simulink model "albedo_test"  (R2023a)
settings: Solver=ode45  StartTime=0.0  StopTime=5.0  RelTol=1e-3  EnableMultiTasking=on
libraries: aausat3_lib x19
settings Model: Creator=kasperv  LastModifiedBy=jacobel-omar
settings SolverCC: AlgebraicLoopSolver=TrustRegion
settings DataIOCC: LimitDataPoints=on  SaveFormat=Array  SignalLoggingSaveFormat=ModelDataLogs  ReturnWorkspaceOutputs=off
settings OptimizationCC: ExpressionDepthLimit=2147483647  LifeSpan=inf
settings DebuggingCC: UnderspecifiedInitializationDetection=Classic  MergeDetectMultiDrivingBlocksExec=none  SolverPrmCheckMsg=warning  FcnCallInpInsideContextMsg=warning  UnconnectedInputMsg=warning  UnconnectedOutputMsg=warning  UnconnectedLineMsg=warning  StateNameClashWarn=warning  SFUnexpectedBacktrackingDiag=warning  SFNoUnconditionalDefaultTransitionDiag=warning  SFExecutionAtInitializationDiag=none  ArithmeticOperatorsInVariantConditions=warning
settings HardwareCC: ProdBitPerPointer=32  ProdBitPerSizeT=32  ProdBitPerPtrDiffT=32  ProdLargestAtomicFloat=None  ProdIntDivRoundTo=Undefined  ProdEndianess=Unspecified  ProdWordSize=32  ProdHWDeviceType=32-bit Generic
settings ModelReferenceCC: PropagateSignalLabelsOutOfModel=off
settings SFSimCC: SimUseLocalCustomCode=off  CustomCodeUndefinedFunction=UseInterfaceOnly
settings RTWCC: RTWUseLocalCustomCode=off
settings CodeAppCC: StateflowObjectComments=on
settings GRTTargetCC: TargetLangStandard=C89/C90 (ANSI)  CombineOutputUpdateFcns=off  GRTInterface=on
settings ConfigComp: CovMetricSettings=dw  CovSaveCumulativeToWorkspaceVar=on  CovSaveSingleToWorkspaceVar=on  CovExternalEMLEnable=off

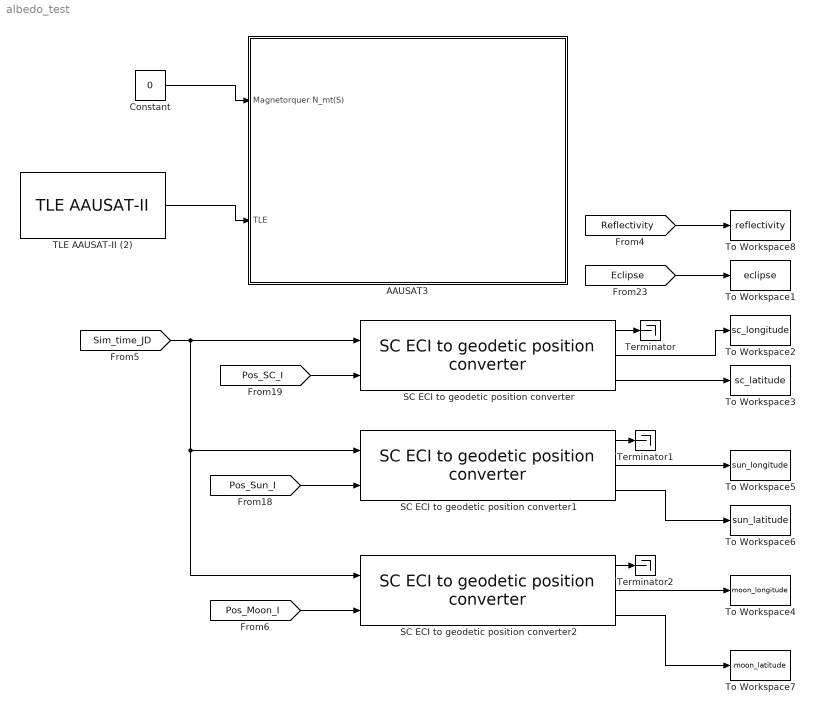
== system albedo_test ==
  AAUSAT3 : Subsystem  AncestorBlock=aausat3_lib/AAUSAT3  mask{r_com_s=[0.0493,0.0972,0.0549], sat_temp_start=293.15, mass_sc=0.7924, Dim=[0.1,0.2,0.1], inertia_c=[0.0017,0.0035,0.0036], init_jd=0, q_s_c=[0 0 0 1], q_init_I_S=[0 0 0 1], w_init_s=[0.1,0.1,0.1], Cd=2, rho=3.614e-14, solar_m_flux=4.5565e-6, solar_absorb_coeff=1.5, theta_e=65, refldata=load('lib/AlbedoToolbox-1.0/refl_data/2005/ga050101-051231'), redfac=1, Ts=1, enable_sensor_emulation=on, enable_env_disturbance=off}
      mask prompts: r_com_s "Center of Mass:"; sat_temp_start "Start Temperature of the Satellite [K]:"; mass_sc "Mass of the Satellite [kg]:"; Dim "Dimension of the Satellite [x,y,z][m];"; inertia_c "Inertia Matrix of the Satellite:"; init_jd "Initial time [JD]:"; q_s_c "Controller Reference Frame (S->C):"; q_init_I_S "Initial Attitude (I->S):"; w_init_s "Initial Angular Rate (S):"; Cd "Atmospheric Drag Coefficient [-]:"; rho "Atmospheric Density [kg/m^3]:"; solar_m_flux "Solar Momentum Flux [kg/ms^2]:"; solar_absorb_coeff "Solar Absorbtion Coefficient [-]:"; theta_e "Max. Angle of Theta [deg](eclipse: theta>r_earth/norm(R_SA)):"; refldata "Reflectivity Data (REFL Struct):"; redfac "Reduction Factor:"; Ts "Albedo Sampling Time [s]:"; enable_sensor_emulation "Enable Sensor Emulation."; enable_env_disturbance "Enable Environment Disturbance."
      mask Display:
      | image(imread('sat.jpg'));
      | color('w');
      | port_label('input', 1, 'N_mt(S)');
      | port_label('input', 2, 'TLE');
  Constant : Constant  Value=0
  SC ECI to geodetic position converter : aausat3_lib/Other Model Utilities/SC ECI to geodetic position converter
      settings: SourceProductName=AAUSAT3
  SC ECI to geodetic position converter1 : aausat3_lib/Other Model Utilities/SC ECI to geodetic position converter
      settings: SourceProductName=AAUSAT3
  SC ECI to geodetic position converter2 : aausat3_lib/Other Model Utilities/SC ECI to geodetic position converter
      settings: SourceProductName=AAUSAT3
  TLE AAUSAT-II (2) : aausat3_lib/Orbit and Ephemeris/TLE AAUSAT-II  satname='AAUSAT-II'  JulianDay=09321.69542252  xndt2o=0.00000555  xndd6o=0.0  bstar=.76898e-4  xincl=97.9251  xnodeo=24.1597  eo=0.0014245  omegao=254.1774  xmo=105.7862  xno=14.81823818  ts=1
      settings: SourceProductName=AAUSAT3
  Terminator : Terminator
  Terminator1 : Terminator
  Terminator2 : Terminator
  To Workspace1 : ToWorkspace  VariableName=eclipse  SampleTime=1
  To Workspace2 : ToWorkspace  VariableName=sc_longitude  SampleTime=1
  To Workspace3 : ToWorkspace  VariableName=sc_latitude  SampleTime=1
  To Workspace4 : ToWorkspace  VariableName=moon_longitude  SampleTime=1
  To Workspace5 : ToWorkspace  VariableName=sun_longitude  SampleTime=1
  To Workspace6 : ToWorkspace  VariableName=sun_latitude  SampleTime=1
  To Workspace7 : ToWorkspace  VariableName=moon_latitude  SampleTime=1
  To Workspace8 : ToWorkspace  VariableName=reflectivity  SampleTime=1
  wires:
  TLE AAUSAT-II (2)/1 -> AAUSAT3/2(TLE)
  Constant/1 -> AAUSAT3/1(Magnetorquer N_mt(S))
  [Eclipse] -> To Workspace1/1
  [Sim_time_JD] -> SC ECI to geodetic position converter/1, SC ECI to geodetic position converter1/1, SC ECI to geodetic position converter2/1
  [Pos_SC_I] -> SC ECI to geodetic position converter/2
  [Pos_Sun_I] -> SC ECI to geodetic position converter1/2
  SC ECI to geodetic position converter/1 -> Terminator/1
  SC ECI to geodetic position converter/2 -> To Workspace2/1
  SC ECI to geodetic position converter/3 -> To Workspace3/1
  SC ECI to geodetic position converter1/3 -> To Workspace6/1
  SC ECI to geodetic position converter1/2 -> To Workspace5/1
  SC ECI to geodetic position converter1/1 -> Terminator1/1
  [Pos_Moon_I] -> SC ECI to geodetic position converter2/2
  SC ECI to geodetic position converter2/3 -> To Workspace7/1
  SC ECI to geodetic position converter2/2 -> To Workspace4/1
  SC ECI to geodetic position converter2/1 -> Terminator2/1
  [Reflectivity] -> To Workspace8/1

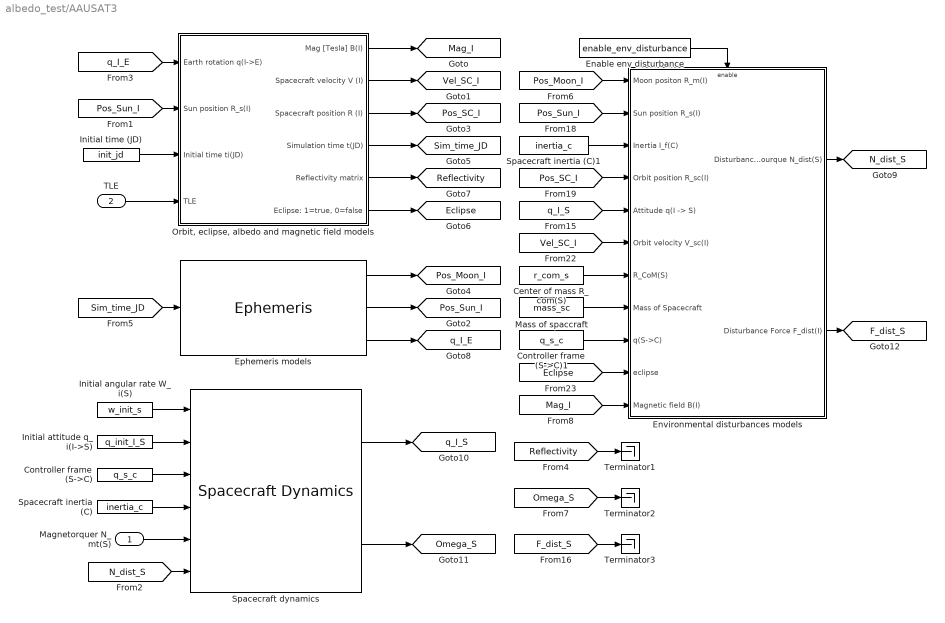
== system albedo_test/AAUSAT3 ==
  Magnetorquer N_mt(S) : Inport
  TLE : Inport  Port=2
  Center of mass R_com(S) : Constant  Value=r_com_s
  Controller frame (S->C) : Constant  Value=q_s_c
  Controller frame (S->C)1 : Constant  Value=q_s_c
  Enable env disturbance : Constant  Value=enable_env_disturbance
  Environmental disturbances models : Subsystem  AncestorBlock=aausat3_lib/Disturbances/Environment Disturbances  mask{Dim=Dim, sola_m_flux=solar_m_flux, solar_absorb_coeff=solar_absorb_coeff, rho=rho, Cd=Cd, G=6.672e-11, M_sun=1.989e30, M_earth=5.9742e24, M_moon=0.073483e24, enable_rad_dist=on, enable_atmospheric_dist=on, enable_gravity_dist=on, enable_mag_residual_dist=on}
      mask prompts: Dim "Satellite Dimension [x,y,z][m]:"; sola_m_flux "Solar Momentum Flux [kg/ms^2]:"; solar_absorb_coeff "Solar Absorbtion Coefficient [-]:"; rho "Atmospheric Density [kg/m^3]:"; Cd "Atmospheric Drag Coefficient [-]:"; G "Gravitational Constant [m^3/kgs^2]:"; M_sun "Mass of the Sun [kg]:"; M_earth "Mass of the Earth [kg]:"; M_moon "Mass of the Moon [kg]:"; enable_rad_dist "Enable Radiation Disturbanceses."; enable_atmospheric_dist "Enable Atmospheric Disturbanceses."; enable_gravity_dist "Enable Gravity Disturbanceses."; enable_mag_residual_dist "Enable Magnetic Residual Disturbance"
      mask help: Torque and force from the environment affecting the satellite.
  Ephemeris models : aausat3_lib/Orbit and Ephemeris/Ephemeris  SystemSampleTime=-1  VariantActivationTime=update diagram  Latency=0  AutoFrameSizeCalculation=off
      settings: SourceProductName=AAUSAT3
  Initial angular rate W_i(S) : Constant  Value=w_init_s
  Initial attitude q_i(I->S) : Constant  Value=q_init_I_S
  Initial time (JD) : Constant  Value=init_jd
  Mass of spaccraft : Constant  Value=mass_sc
  "Orbit, eclipse, albedo and magnetic field models" : Subsystem  AncestorBlock=aausat3_lib/Orbit and Ephemeris/Orbit and Magnetic field models  mask{r_e=6371e3, theta_e=theta_e, refldata=refldata, redfac=redfac, Ts=Ts, enable_eclipse=on, enable_IGRF=on, reflectivity_enabled=off, enable_sgp4=on, enable_custom_time=on}
      mask prompts: r_e "Radius of the Earth [m]:"; theta_e "Max. Angle of Theta [deg] (eclipse: theta > r_earth/norm(R_SA)):"; refldata "Reflectivity Data (REFL Struct):"; redfac "Reduction Factor:"; Ts "Albedo Model Sampling Time [s]:"; enable_eclipse "Enable Eclipse Model."; enable_IGRF "Enable IGRF Model."; reflectivity_enabled "Enable Albedo Model."; enable_sgp4 "Enable SGP4 Model."; enable_custom_time "Enable Custom Time."
      mask help: When you want to use "Other" make sure to define the TLE in the SGP4 subsystem.
  Spacecraft dynamics : aausat3_lib/Dynamics and Kinematics/Spacecraft Dynamics  SystemSampleTime=-1  VariantActivationTime=update diagram  Latency=0  AutoFrameSizeCalculation=off
      settings: SourceProductName=AAUSAT3
  Spacecraft inertia (C) : Constant  Value=inertia_c
  Spacecraft inertia (C)1 : Constant  Value=inertia_c
  Terminator1 : Terminator
  Terminator2 : Terminator
  Terminator3 : Terminator
  tag scope: Eclipse=global, F_dist_S=global, Mag_I=global, N_dist_S=global, Omega_S=global, Pos_Moon_I=global, Pos_SC_I=global, Pos_Sun_I=global, Reflectivity=global, Sim_time_JD=global, Vel_SC_I=global, q_I_E=global, q_I_S=global
  wires:
  [q_I_S] -> Environmental disturbances models/5("Attitude q(I -> S)")
  Environmental disturbances models/2(Disturbance Force F_dist(I)) -> [F_dist_S]
  Environmental disturbances models/1(Disturbance tourque N_dist(S)) -> [N_dist_S]
  [Mag_I] -> Environmental disturbances models/11(Magnetic field B(I))
  [Eclipse] -> Environmental disturbances models/10(eclipse)
  Controller frame (S->C)1/1 -> Environmental disturbances models/9(q(S->C))
  Mass of spaccraft/1 -> Environmental disturbances models/8(Mass of Spacecraft)
  Center of mass R_com(S)/1 -> Environmental disturbances models/7(R_CoM(S))
  [Vel_SC_I] -> Environmental disturbances models/6(Orbit velocity V_sc(I))
  [Pos_SC_I] -> Environmental disturbances models/4(Orbit position R_sc(I))
  Spacecraft inertia (C)1/1 -> Environmental disturbances models/3(Inertia I_f(C))
  [Pos_Sun_I] -> Environmental disturbances models/2(Sun position R_s(I))
  Enable env disturbance/1 -> Environmental disturbances models/Enable
  [Pos_Moon_I] -> Environmental disturbances models/1(Moon positon R_m(I))
  TLE/1 -> "Orbit, eclipse, albedo and magnetic field models"/4(TLE)
  [q_I_E] -> "Orbit, eclipse, albedo and magnetic field models"/1(Earth rotation q(I->E))
  [Omega_S] -> Terminator2/1
  [Reflectivity] -> Terminator1/1
  Initial time (JD)/1 -> "Orbit, eclipse, albedo and magnetic field models"/3(Initial time ti(JD))
  [Pos_Sun_I] -> "Orbit, eclipse, albedo and magnetic field models"/2(Sun position R_s(I))
  Spacecraft dynamics/1 -> [q_I_S]
  [F_dist_S] -> Terminator3/1
  "Orbit, eclipse, albedo and magnetic field models"/6("Eclipse: 1=true, 0=false") -> [Eclipse]
  Magnetorquer N_mt(S)/1 -> Spacecraft dynamics/5
  "Orbit, eclipse, albedo and magnetic field models"/1(Mag [Tesla] B(I)) -> [Mag_I]
  "Orbit, eclipse, albedo and magnetic field models"/2(Spacecraft velocity V (I)) -> [Vel_SC_I]
  Spacecraft inertia (C)/1 -> Spacecraft dynamics/4
  Controller frame (S->C)/1 -> Spacecraft dynamics/3
  "Orbit, eclipse, albedo and magnetic field models"/3(Spacecraft position R (I)) -> [Pos_SC_I]
  Initial angular rate W_i(S)/1 -> Spacecraft dynamics/1
  Initial attitude q_i(I->S)/1 -> Spacecraft dynamics/2
  "Orbit, eclipse, albedo and magnetic field models"/4(Simulation time t(JD)) -> [Sim_time_JD]
  Ephemeris models/1 -> [Pos_Moon_I]
  Ephemeris models/2 -> [Pos_Sun_I]
  Ephemeris models/3 -> [q_I_E]
  "Orbit, eclipse, albedo and magnetic field models"/5(Reflectivity matrix) -> [Reflectivity]
  Spacecraft dynamics/2 -> [Omega_S]
  [Sim_time_JD] -> Ephemeris models/1
  [N_dist_S] -> Spacecraft dynamics/6

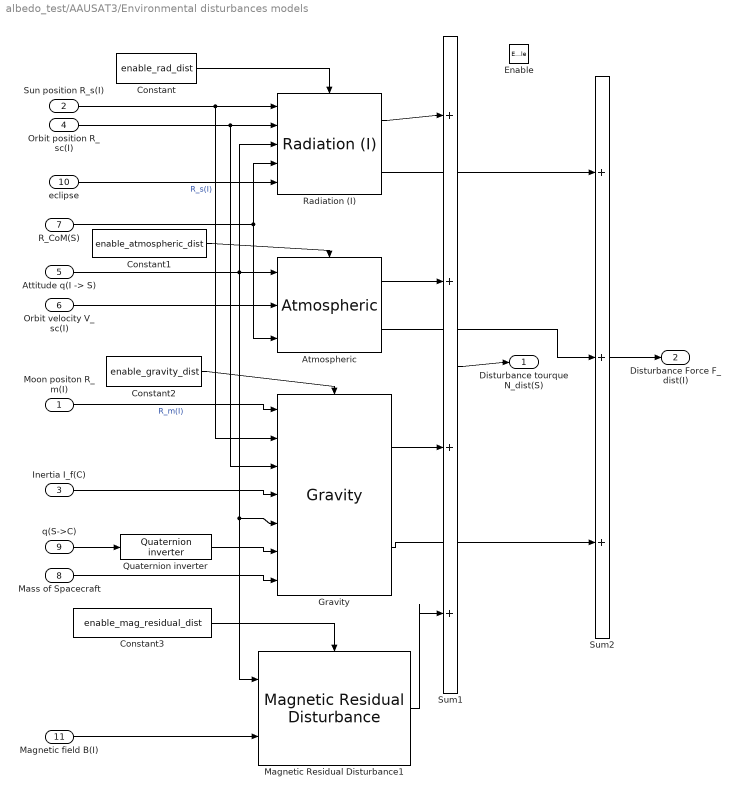
== system albedo_test/AAUSAT3/Environmental disturbances models ==
  Moon positon R_m(I) : Inport
  Sun position R_s(I) : Inport  Port=2
  Inertia I_f(C) : Inport  Port=3
  Orbit position R_sc(I) : Inport  Port=4
  "Attitude q(I -> S)" : Inport  Port=5
  Orbit velocity V_sc(I) : Inport  Port=6
  R_CoM(S) : Inport  Port=7
  Mass of Spacecraft : Inport  Port=8
  q(S->C) : Inport  Port=9
  eclipse : Inport  Port=10
  Magnetic field B(I) : Inport  Port=11
  Enable : EnablePort
  Atmospheric : aausat3_lib/Disturbances/Atmospheric  Dim=Dim  Cd=Cd  rho=rho
      settings: SourceProductName=AAUSAT3
  Constant : Constant  Value=enable_rad_dist
  Constant1 : Constant  Value=enable_atmospheric_dist
  Constant2 : Constant  Value=enable_gravity_dist
  Constant3 : Constant  Value=enable_mag_residual_dist
  Gravity : aausat3_lib/Disturbances/Gravity  G=G  M_sun=M_sun  M_moon=M_moon  M_earth=M_earth  enable_moon_G=off  enable_sun_G=off  enable_zharm_earth=off  enable_gravity_torque=on
      link override Gravity Gradient Torque: G=G  M_earth=M_earth
      settings: SourceProductName=AAUSAT3
  Magnetic Residual Disturbance1 : aausat3_lib/Disturbances/Magnetic Residual Disturbance  mag_moment=0.001
      settings: SourceProductName=AAUSAT3
  Quaternion inverter : aausat3_lib/Math Utilities/Quaternion operations/Quaternion inverter  SystemSampleTime=-1  VariantActivationTime=update diagram  Latency=0  AutoFrameSizeCalculation=off
      settings: SourceProductName=AAUSAT3
  Radiation (I) : aausat3_lib/Disturbances/Radiation (I)  Dim=Dim  solar_m_flux=solar_m_flux  solar_absorb_coeff=solar_absorb_coeff
      settings: SourceProductName=AAUSAT3
  Sum1 : Sum  Inputs=++++  SaturateOnIntegerOverflow=on
  Sum2 : Sum  Inputs=+++  SaturateOnIntegerOverflow=on
  Disturbance tourque N_dist(S) : Outport
  Disturbance Force F_dist(I) : Outport  Port=2
  wires:
  Inertia I_f(C)/1 -> Gravity/4
  eclipse/1 -> Radiation (I)/5
  Sum2/1 -> Disturbance Force F_dist(I)/1
  Sum1/1 -> Disturbance tourque N_dist(S)/1
  Gravity/2 -> Sum2/3
  Radiation (I)/2 -> Sum2/1
  Gravity/1 -> Sum1/3
  Atmospheric/1 -> Sum1/2
  Orbit velocity V_sc(I)/1 -> Atmospheric/2
  Orbit position R_sc(I)/1 -> Radiation (I)/2, Gravity/3
  "Attitude q(I -> S)"/1 -> Radiation (I)/3, Atmospheric/1, Magnetic Residual Disturbance1/1, Gravity/5
  Sun position R_s(I)/1 -> Radiation (I)/1, Gravity/2  "R_s(I)"
  Moon positon R_m(I)/1 -> Gravity/1  "R_m(I)"
  Mass of Spacecraft/1 -> Gravity/7
  Quaternion inverter/1 -> Gravity/6
  q(S->C)/1 -> Quaternion inverter/1
  R_CoM(S)/1 -> Radiation (I)/4, Atmospheric/3
  Constant/1 -> Radiation (I)/Enable
  Constant2/1 -> Gravity/Enable
  Constant1/1 -> Atmospheric/Enable
  Constant3/1 -> Magnetic Residual Disturbance1/Enable
  Radiation (I)/1 -> Sum1/1
  Atmospheric/2 -> Sum2/2
  Magnetic Residual Disturbance1/1 -> Sum1/4
  Magnetic field B(I)/1 -> Magnetic Residual Disturbance1/2

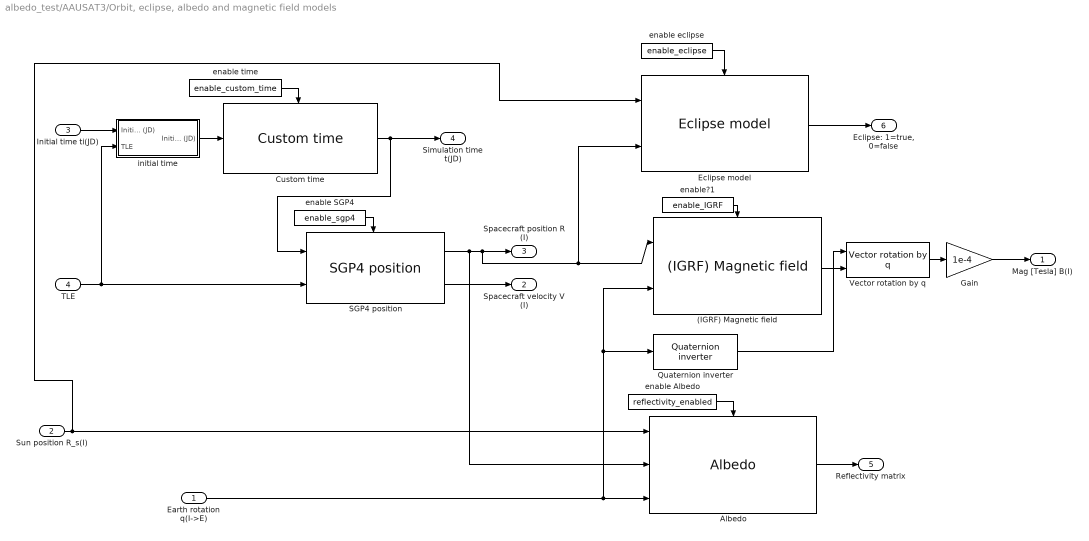
== system albedo_test/AAUSAT3/Orbit, eclipse, albedo and magnetic field models ==
  Earth rotation q(I->E) : Inport
  Sun position R_s(I) : Inport  Port=2
  Initial time ti(JD) : Inport  Port=3
  TLE : Inport  Port=4
  (IGRF) Magnetic field : aausat3_lib/Orbit and Ephemeris/(IGRF) Magnetic field  SystemSampleTime=-1  VariantActivationTime=update diagram  Latency=0  AutoFrameSizeCalculation=off
      settings: SourceProductName=AAUSAT3
  Albedo : aausat3_lib/Orbit and Ephemeris/Albedo  refldata=refldata  redfac=redfac  Ts=Ts
      settings: SourceProductName=AAUSAT3
  Custom time : aausat3_lib/Orbit and Ephemeris/Custom time  SystemSampleTime=-1  VariantActivationTime=update diagram  Latency=0  AutoFrameSizeCalculation=off
      settings: SourceProductName=AAUSAT3
  Eclipse model : aausat3_lib/Orbit and Ephemeris/Eclipse model  r_e=r_e  enable=off  theta_e=theta_e
      settings: SourceProductName=AAUSAT3
  Gain : Gain  Gain=1e-4
  Quaternion inverter : aausat3_lib/Math Utilities/Quaternion operations/Quaternion inverter  SystemSampleTime=-1  VariantActivationTime=update diagram  Latency=0  AutoFrameSizeCalculation=off
      settings: SourceProductName=AAUSAT3
  SGP4 position : aausat3_lib/Orbit and Ephemeris/SGP4 position  SystemSampleTime=-1  VariantActivationTime=update diagram  Latency=0  AutoFrameSizeCalculation=off
      settings: SourceProductName=AAUSAT3
  Vector rotation by q : aausat3_lib/Math Utilities/Quaternion operations/Vector rotation by q  SystemSampleTime=-1  VariantActivationTime=update diagram  Latency=0  AutoFrameSizeCalculation=off
      settings: SourceProductName=AAUSAT3
  enable Albedo : Constant  Value=reflectivity_enabled
  enable SGP4 : Constant  Value=enable_sgp4
  enable eclipse : Constant  Value=enable_eclipse
  enable time : Constant  Value=enable_custom_time
  enable?1 : Constant  Value=enable_IGRF
  initial time : Subsystem
  Mag [Tesla] B(I) : Outport
  Spacecraft velocity V (I) : Outport  Port=2
  Spacecraft position R (I) : Outport  Port=3
  Simulation time t(JD) : Outport  Port=4
  Reflectivity matrix : Outport  Port=5
  "Eclipse: 1=true, 0=false" : Outport  Port=6  PortDimensions=1
  wires:
  Eclipse model/1 -> "Eclipse: 1=true, 0=false"/1
  enable Albedo/1 -> Albedo/Enable
  enable?1/1 -> (IGRF) Magnetic field/Enable
  Vector rotation by q/1 -> Gain/1
  Quaternion inverter/1 -> Vector rotation by q/1
  enable time/1 -> Custom time/Enable
  Custom time/1 -> Simulation time t(JD)/1, SGP4 position/1
  Albedo/1 -> Reflectivity matrix/1
  Sun position R_s(I)/1 -> Eclipse model/1, Albedo/1
  Earth rotation q(I->E)/1 -> (IGRF) Magnetic field/2, Quaternion inverter/1, Albedo/3
  enable SGP4/1 -> SGP4 position/Enable
  SGP4 position/1 -> (IGRF) Magnetic field/1, Eclipse model/2, Spacecraft position R (I)/1, Albedo/2
  SGP4 position/2 -> Spacecraft velocity V (I)/1
  (IGRF) Magnetic field/1 -> Vector rotation by q/2
  Gain/1 -> Mag [Tesla] B(I)/1
  enable eclipse/1 -> Eclipse model/Enable
  TLE/1 -> SGP4 position/2, initial time/2(TLE)
  initial time/1(Initial time out (JD)) -> Custom time/1
  Initial time ti(JD)/1 -> initial time/1(Initial time in (JD))

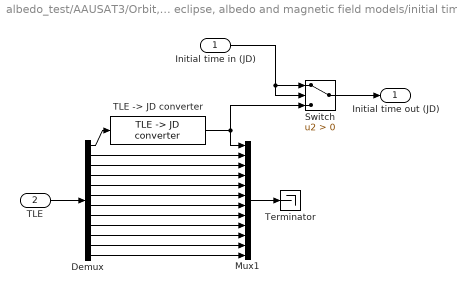
== system albedo_test/AAUSAT3/Orbit, eclipse, albedo and magnetic field models/initial time ==
  Initial time in (JD) : Inport
  TLE : Inport  Port=2
  Demux : Demux  Outputs=12
  Mux1 : Mux  Inputs=12
  Switch : Switch  Criteria=u2 > Threshold  SaturateOnIntegerOverflow=off  InputSameDT=off
  "TLE -> JD converter" : aausat3_lib/Other Model Utilities/TLE -> JD converter  SystemSampleTime=-1  VariantActivationTime=update diagram  Latency=0  AutoFrameSizeCalculation=off
      settings: SourceProductName=AAUSAT3
  Terminator : Terminator
  Initial time out (JD) : Outport
  wires:
  "TLE -> JD converter"/1 -> Mux1/1, Switch/3
  Demux/1 -> "TLE -> JD converter"/1
  Demux/12 -> Mux1/12
  Demux/11 -> Mux1/11
  Demux/10 -> Mux1/10
  Demux/9 -> Mux1/9
  Demux/8 -> Mux1/8
  Demux/7 -> Mux1/7
  Demux/6 -> Mux1/6
  Demux/5 -> Mux1/5
  Demux/4 -> Mux1/4
  Demux/3 -> Mux1/3
  Demux/2 -> Mux1/2
  TLE/1 -> Demux/1
  Initial time in (JD)/1 -> Switch/2, Switch/1
  Switch/1 -> Initial time out (JD)/1
  Mux1/1 -> Terminator/1
